simulink model "REDIS_model"  (R2024a)
settings: Solver=FixedStepDiscrete  StartTime=0.0  StopTime=10  FixedStep=1  RelTol=1e-3  EnableMultiTasking=on
InitFcn:
  | redis_datatypes;
values from neighbouring files (symbols this model uses):
  redis_hostname = [uint8(address) 0]    [redis_datatypes.m]
  redis_port = [uint8('6379') 0]    [redis_datatypes.m]
settings Model: ModifiedByFormat=Sun Aug 30 12:23:04 2015  Creator=Castorp  LastModifiedBy=Sun Aug 30 12:23:04 2015
settings Model: ModifiedHistory=|
  | Example of REDIS connector implemented as a S-Function
  | 
  | 
  | Castorp. <cidart@gmail.com>
settings SolverCC: AlgebraicLoopSolver=TrustRegion
settings DataIOCC: LimitDataPoints=on  SaveFormat=Structure  SignalLoggingSaveFormat=ModelDataLogs  SaveOutput=off  SignalLogging=off  SaveTime=off  ReturnWorkspaceOutputs=off
settings OptimizationCC: LifeSpan=Inf  EfficientTunableParamExpr=on
settings DebuggingCC: SolverPrmCheckMsg=warning  MultiTaskDSMMsg=warning  MultiTaskCondExecSysMsg=none  UnconnectedInputMsg=warning  UnconnectedOutputMsg=warning  UnconnectedLineMsg=warning  SFUnexpectedBacktrackingDiag=warning  SFNoUnconditionalDefaultTransitionDiag=warning  SFExecutionAtInitializationDiag=none  ArithmeticOperatorsInVariantConditions=warning
settings HardwareCC: ProdBitPerLong=64  ProdHWDeviceType=Apple->ARM64  TargetIntDivRoundTo=Zero  TargetEndianess=LittleEndian  TargetHWDeviceType=Intel->x86/Pentium
settings ModelReferenceCC: PropagateSignalLabelsOutOfModel=off
settings SFSimCC: SimCustomHeaderCode="#include \"REDIS_custom.h\""  SimUserIncludeDirs=hiredis  SimUserLibraries=libhiredis.a  SimUseLocalCustomCode=off  MATLABDynamicMemAlloc=off  CustomCodeUndefinedFunction=UseInterfaceOnly  SimTargetLang=C++
settings SFSimCC: SimUserSources=|
  | REDIS_wrapper.cpp
  | REDIS_custom.cpp
settings RTWCC: Description=Embedded Coder  SystemTargetFile=ert.tlc  GenCodeOnly=on  TemplateMakefile=ert_default_tmf  GenerateReport=on  RetainRTWFile=on  RTWUseLocalCustomCode=off  RTWUseSimCustomCode=on  CustomHeaderCode="#include \"REDIS_custom.h\""  CustomInclude=hiredis  CustomLibrary=libhiredis.a  IncludeHyperlinkInReport=on  LaunchReport=on  TargetLang=C++  GPUComputeCapability=3.5
settings RTWCC: CustomSource=|
  | REDIS_wrapper.cpp
  | REDIS_custom.cpp
settings CodeAppCC: IgnoreCustomStorageClasses=off  StateflowObjectComments=on
settings ERTTargetCC: MultiwordLength=2048  GenerateSampleERTMain=on  SupportAbsoluteTime=off  SupportComplex=off  SupportVariableSizeSignals=on  ERTCustomFileTemplate=example_file_process.tlc  ConvertIfToSwitch=off  SuppressUnreachableDefaultCases=off
settings ConfigComp: CovMetricSettings=dw  CovSaveCumulativeToWorkspaceVar=on  CovSaveSingleToWorkspaceVar=on  CovExternalEMLEnable=off

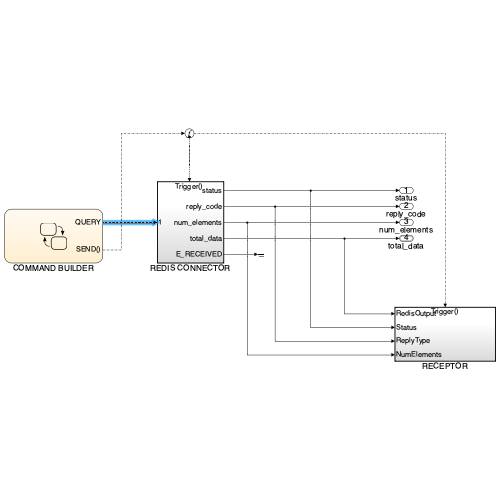
[thumbnail: Simulink's stored preview of the top-level diagram]
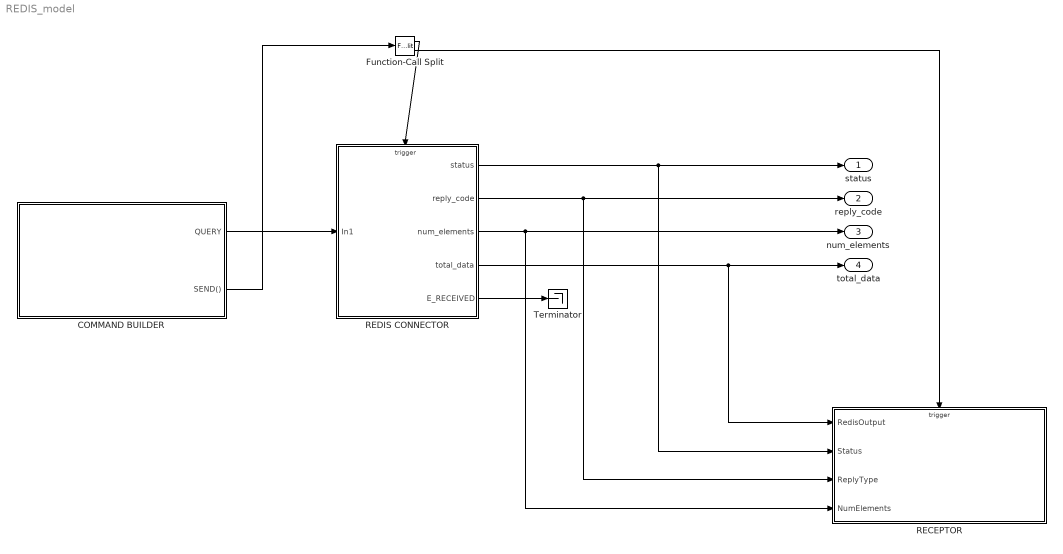
== system REDIS_model ==
  COMMAND BUILDER : Stateflow chart  TreatAsAtomicUnit=on
  Function-Call Split : FunctionCallSplit  NumOutputPorts=2
  RECEPTOR : Subsystem  TreatAsAtomicUnit=on
  "REDIS CONNECTOR " : Subsystem  TreatAsAtomicUnit=on
  Terminator : Terminator
  status : Outport
  reply_code : Outport  Port=2
  num_elements : Outport  Port=3
  total_data : Outport  Port=4  OutDataTypeStr=Bus: RedisValue
  wires:
  COMMAND BUILDER/1(QUERY) -> "REDIS CONNECTOR "/1(In1)
  "REDIS CONNECTOR "/2(reply_code) -> RECEPTOR/3(ReplyType), reply_code/1
  "REDIS CONNECTOR "/3(num_elements) -> num_elements/1, RECEPTOR/4(NumElements)
  "REDIS CONNECTOR "/1(status) -> status/1, RECEPTOR/2(Status)
  "REDIS CONNECTOR "/4(total_data) -> total_data/1, RECEPTOR/1(RedisOutput)
  COMMAND BUILDER/2(SEND()) -> Function-Call Split/1
  Function-Call Split/2 -> RECEPTOR/Trigger
  Function-Call Split/1 -> "REDIS CONNECTOR "/Trigger
  "REDIS CONNECTOR "/5(E_RECEIVED) -> Terminator/1

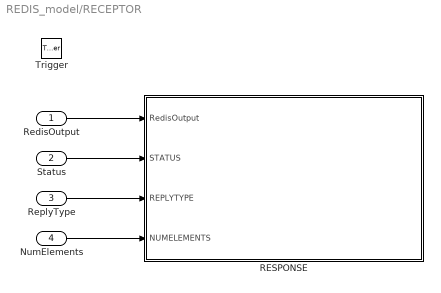
== system REDIS_model/RECEPTOR ==
  RedisOutput : Inport
  Status : Inport  Port=2
  ReplyType : Inport  Port=3
  NumElements : Inport  Port=4
  Trigger : TriggerPort  TriggerType=function-call  VariantControl=(inherit)
  RESPONSE : Stateflow chart  TreatAsAtomicUnit=on
  wires:
  RedisOutput/1 -> RESPONSE/1(RedisOutput)
  Status/1 -> RESPONSE/2(STATUS)
  ReplyType/1 -> RESPONSE/3(REPLYTYPE)
  NumElements/1 -> RESPONSE/4(NUMELEMENTS)

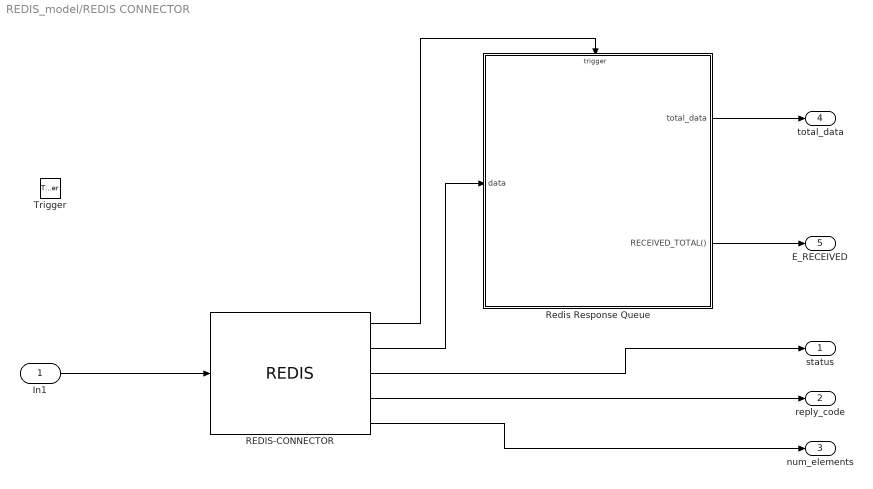
== system REDIS_model/REDIS CONNECTOR  ==
  In1 : Inport
  Trigger : TriggerPort  TriggerType=function-call  VariantControl=(inherit)
  REDIS-CONNECTOR : S-Function  FunctionName=REDIS  Parameters=redis_hostname,redis_port  SFunctionDeploymentMode=off  EnableBusSupport=off
  Redis Response Queue : Stateflow chart  TreatAsAtomicUnit=on
  status : Outport  InitialOutput=-1
  reply_code : Outport  Port=2  InitialOutput=0
  num_elements : Outport  Port=3  InitialOutput=0
  total_data : Outport  Port=4  OutDataTypeStr=Bus: RedisValue  InitialOutput=0
  E_RECEIVED : Outport  Port=5
  wires:
  In1/1 -> REDIS-CONNECTOR/1
  REDIS-CONNECTOR/2 -> Redis Response Queue/1(data)
  REDIS-CONNECTOR/1 -> Redis Response Queue/Trigger
  REDIS-CONNECTOR/3 -> status/1
  REDIS-CONNECTOR/4 -> reply_code/1
  REDIS-CONNECTOR/5 -> num_elements/1
  Redis Response Queue/1(total_data) -> total_data/1
  Redis Response Queue/2(RECEIVED_TOTAL()) -> E_RECEIVED/1

== stateflow chart REDIS_model/REDIS CONNECTOR /Redis Response Queue ==
  state STARTED
    en:
    printf('Starting transfer, reseting Queue!\n');
    resetQueue();
  state FULL
    en:
    buildOutput();
    printf('REDIS Response Queue FULL with %0.f elements\n',counter);
    %send(FULL);
    send(RECEIVED_TOTAL);
    du:
    printf('IGNORED redis value sent to Queue (Queue FULL)\n');
  state RECEIVED
    en:
    printf('RECEIVED Single Redis Value in Queue!\n');
    printRedisSingleValue();
    storeData();
    du:
    printf('RECEIVED Single Redis Value in Queue!\n');
    printRedisSingleValue();
    storeData();
  state FINISHED
    en:
    buildOutput();
    send(RECEIVED_TOTAL);
  (default) -> (junction 40)
  STARTED -> (junction 40)
  (junction 40) -> STARTED [order 3] : STARTED
  (junction 40) -> FINISHED [order 2] : FINISHED
  (junction 40) -> (junction 23) [order 1] : RECEIVED_SINGLE
  (junction 37) -> (junction 40)
  (junction 23) -> RECEIVED [order 1] : [counter <= (capacity-1)]
      | {counter = counter + 1;}
  (junction 23) -> FULL [order 2]
  FINISHED -> (junction 37)
  RECEIVED -> (junction 37)
  FULL -> FINISHED : FINISHED
  data: data input uint8 size=255; total_data output Bus: RedisValue size=capacity; capacity constant double size=1 =numOutputs; counter local double size=1 =0; numOutputs parameter double
  data capacity settings: description=Queue capacity
  events: RECEIVED_SINGLE input FUNCTION_CALL_EVENT; FINISHED input FUNCTION_CALL_EVENT; RECEIVED_TOTAL output FUNCTION_CALL_EVENT; STARTED input FUNCTION_CALL_EVENT
  function printRedisSingleValue:
    | function printRedisSingleValue()
    | %#codegen
    | 
    | 
    | fprintf('-> Received Redis Value (length:%d): "%s"\n',int32(length(char(data))),char(data));
    | 
    | 
    | end
  function buildOutput:
    | function buildOutput
    | 
    | fprintf('DATA TRANSFER FINISHED!\n');
    | 
    | end
  function storeData:
    | function storeData
    | 
    | 
    | total_data(counter).value = data;
    | 
    | 
    | end
  function resetQueue:
    | function resetQueue
    |  
    | counter = 0;
    | 
    | len = numel(total_data);
    | for i=1:len
    |     total_data(i).value = zeros(255,1,'uint8');
    | end
    | 
    | end

== stateflow chart REDIS_model/COMMAND BUILDER ==
  state EXEC
    en: buildCommand();send(SEND);
    du: buildCommand();send(SEND);
  (default) -> EXEC
  data: QUERY output uint8 size=maxCMDLen; maxCMDLen constant double size=1 =255; cmd_index local double =1
  events: SEND output FUNCTION_CALL_EVENT
  function buildCommand:
    | function buildCommand
    | %#codegen
    | 
    | %CMD
    | %PARAMS
    | num_commands = 8;
    | randn()
    | cmd_struct.cmd = zeros(1,maxCMDLen,'uint8');
    | command = repmat(cmd_struct ,1,num_commands);
    | QUERY = zeros(maxCMDLen,1,'uint8');
    | 
    | % SET keys commands
    | command(1).cmd(1:23)  = uint8('SET EURUSD:last 1.32343');
    | command(2).cmd(1:23)  = uint8('SET GBPJPY:last 186.432');
    | command(3).cmd(1:23)  = uint8('SET AUDUSD:last 0.71882');
    | 
    | % GET keys commands
    | command(4).cmd(1:15)  = uint8('GET EURUSD:last');
    | command(5).cmd(1:15)  = uint8('GET GBPJPY:last');
    | command(6).cmd(1:15)  = uint8('GET AUDUSD:last');
    | 
    | % Push items to list
    | cmd1 = uint8('LPUSH mylist ITEM_1 ITEM_2 ITEM_3 ITEM_4 ITEM_5 ITEM_6 ITEM_7 ITEM_8 ITEM_9 ITEM_10');
    | command(7).cmd(1:length(cmd1)) = cmd1;
    | 
    | % Get list items
    | cmd2 = uint8('LRANGE mylist 0 9');
    | command(8).cmd(1:length(cmd2)) = cmd2;
    | 
    | % Set command index to start
    | if(cmd_index > num_commands)
    |     cmd_index = 1;
    | end
    | 
    | % Get current command
    | current_command = command(cmd_index).cmd;
    | 
    | % Output command
    | QUERY(1:length(current_command),1) = current_command';
    | 
    | % Incr command index.
    | cmd_index = cmd_index + 1;

== stateflow chart REDIS_model/RECEPTOR/RESPONSE ==
  state ERROR
    en: printState();
    du: printState();
  state RECEIVED
    en: printRedisInput(); printState();
    du: printRedisInput(); printState();
    state printRedisInput [function]
      (default) -> (junction 39) : {printResponse(RedisOutput)}
  (default) -> (junction 26)
  (junction 26) -> ERROR [order 2]
  (junction 26) -> RECEIVED [order 1] : [STATUS==0]
  RECEIVED -> ERROR : [STATUS~=0]
  ERROR -> RECEIVED : [STATUS==0]
  data: redis_response_object function_input; RedisOutput input Bus: RedisValue; STATUS input int32 size=1; REPLYTYPE input uint8; NUMELEMENTS input uint32
  function printResponse(redis_response_object):
    | function printResponse(redis_response_object)
    | %#codegen
    |  
    | elements = uint8(numel(redis_response_object));
    | 
    | for i=1:elements    
    |         
    |     val = redis_response_object(i).value';    
    |     if (any(val))
    |         fprintf('total_data element %f: %s\n',single(i),char(val));        
    |     end   
    | end
    | 
    | end
  function printState:
    | function printState
    | %#codegen
    | 
    | fprintf('* REDIS CONNECTOR STATE:\n');
    | fprintf('[x] STATUS: %f -> %s\n',single(STATUS),status_name(STATUS));
    | fprintf('[x] REPLY TYPE: %f -> %s\n',single(REPLYTYPE),replytype_name(REPLYTYPE));
    | fprintf('[x] NUM ELEMENTS: %f\n\n',single(NUMELEMENTS));
    | 
    | 
    | end
    | 
    | function name = status_name(code)
    | 
    |    name = char('UNKNOWN');
    |    switch(code)
    |        case -1
    |            name = char('REDIS_ERR');                  
    |        case 0
    |            name = char('REDIS_OK');           
    |        case 1
    |            name = char('REDIS_ERR_IO');           
    |        case 2
    |            name = char('REDIS_ERR_OTHER');
    |        case 3
    |            name = char('REDIS_ERR_EOF');
    |        case 4
    |            name = char('REDIS_ERR_PROTOCOL');
    |        case 5
    |            name = char('REDIS_ERR_OOM');          
    |    end
    | end
    | 
    | 
    | function name = replytype_name(code)
    | 
    |    name = char('UNKNOWN');
    |    switch(code)        
    |        case 1
    |            name = char('REDIS_REPLY_STRING');           
    |        case 2
    |            name = char('REDIS_REPLY_ARRAY');
    |        case 3
    |            name = char('REDIS_REPLY_INTEGER');
    |        case 4
    |            name = char('REDIS_REPLY_NIL');
    |        case 5
    |            name = char('REDIS_REPLY_STATUS'); 
    |        case 6
    |            name = char('REDIS_REPLY_ERROR');            
    |    end
    | end
